simulink model "a1"  (R2018b)
settings: Solver=FixedStepAuto  StartTime=0.0  StopTime=10.4  FixedStep=0.1  RelTol=1e-3
settings Model: Creator=a4327  LastModifiedBy=a4327

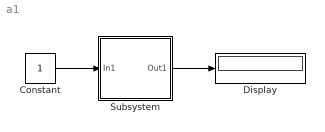
== system a1 ==
  Constant : Constant
  Display : Display
  Subsystem : Subsystem
  wires:
  Constant/1 -> Subsystem/1(In1)
  Subsystem/1(Out1) -> Display/1

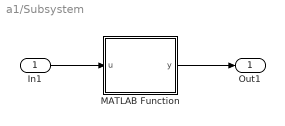
== system a1/Subsystem ==
  In1 : Inport
  MATLAB Function : MATLAB Function  TreatAsAtomicUnit=on
  Out1 : Outport
  wires:
  MATLAB Function/1(y) -> Out1/1
  In1/1 -> MATLAB Function/1(u)

== matlab function a1/Subsystem/MATLAB Function ==
  data: y output; u input
function y=fcn(u)
 global a
% ftest1;
% ftest2;

 y=a;
%  a=y;
%  if a==33
%      a=0;
%  end
end
